simulink model "MBD_W3_P1"  (R2020a)
settings: Solver=VariableStepAuto  StartTime=0.0  StopTime=10.0  RelTol=1e-3
settings Model: Creator=Atri Mondal  LastModifiedBy=Atri Mondal

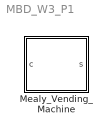
== system MBD_W3_P1 ==
  Mealy_Vending_Machine : Stateflow chart  TreatAsAtomicUnit=on

== stateflow chart MBD_W3_P1/Mealy_Vending_Machine ==
  state got_none
  state nickel
  state dime
  (default) -> got_none
  got_none -> nickel [order 1] : [c==1]{s=0}
  nickel -> got_none [order 2] : [c==2]{s=1}
  dime -> got_none [order 1] : [c==1]{s=1}
  got_none -> dime [order 2] : [c==2]{s=0}
  nickel -> dime [order 1] : [c==1]{s=0}
  dime -> nickel [order 2] : [c==2]{s=1}
  data: c input; s output
